simulink model "OneGFM_V2"  (R2020a)
settings: Solver=VariableStepAuto  StartTime=0.0  StopTime=10  RelTol=1e-6
InitFcn:
  | %initAll
values from neighbouring files (symbols this model uses):
  A_ = A(1:2*Ne,1:2*Ne) - B(1:2*Ne,1:2*Nu)/D(1:2*Nu,1:2*Nu)*C(1:2*Nu,1:2*Ne)    [init_V2.m]
  B_ = B(1:2*Ne,1:2*Nu)/D(1:2*Nu,1:2*Nu)    [init_V2.m]
  C_ = -D(1:2*Nu,1:2*Nu)\C(1:2*Nu,1:2*Ne)    [init_V2.m]
  D_ = inv(D(1:2*Nu,1:2*Nu))    [init_V2.m]
  GFMInit = GFM_init(opdata,GFM_in_gidx,SGFM)    [init_V2.m]
  Nu = length(G_in_gidx)    [init_V2.m]
  RG = gfmdata(:,3)    [GFL_init.m]    (also in GFM_init.m = gfmdata(:,3)./SGFM; GFMparaarea.m = 0; init_V2.m = 1e-06)
  VO = Vm(SG_in_gidx)+(opdata{num2str(SG_in_gidx),2}/1000-1i*opdata{num2str(SG_in_gidx),3}/1000)*RG    [init_V2.m]
  W0 = 2*pi*50    (= 314.159265359)    [GFMparaarea.m]    (also in ONEGFM_analysis.m = 314.1593; init_V2.m)
  X0 = -Adq\Bdq*udq    [init_V2.m]
undefined symbols (not defined in the file or in its folder): full, opdata
libraries: eeTransforms x4, simulink_extras x1
settings Model: Creator=LinSiQi  LastModifiedBy=Qiufan_Yang
settings DebuggingCC: ArithmeticOperatorsInVariantConditions=warning
settings SFSimCC: CustomCodeUndefinedFunction=UseInterfaceOnly
settings CodeAppCC: StateflowObjectComments=on
settings SimscapeCC: SimscapeNormalizeSystem=off

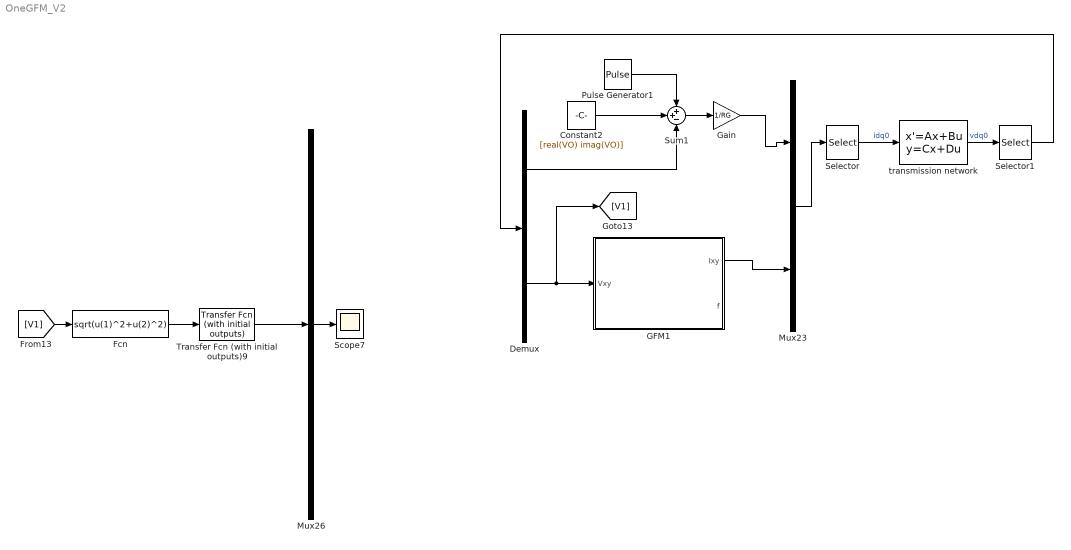
== system OneGFM_V2 ==
  Constant2 : Constant  Value=[real(VO) imag(VO)]
  Demux : Demux  Outputs=2
  Fcn : Fcn  Expr=sqrt(u(1)^2+u(2)^2)
  GFM1 : Subsystem  mask{Pout=opdata{1,2}, Qout=opdata{1,3}, Vout=opdata{1,4}*exp(1i*opdata{1,5}*pi/180), RG=GFMInit.RG(1), LG=GFMInit.LG(1), CF=GFMInit.CF(1), LF=GFMInit.LF(1), RF=GFMInit.RF(1), JGFM=GFMInit.J(1), DGFM=GFMInit.D(1), KPV=GFMInit.KPV(1), KIV=GFMInit.KIV(1), KIF=GFMInit.KIF(1), KPC=GFMInit.KPC(1), KIC=GFMInit.KIC(1), KVF=GFMInit.KVF(1), TVF=GFMInit.TVF(1), Pref=GFMInit.Pref(1), Qref=GFMInit.Qref(1), Vd0=GFMInit.Vd0(1), theta0=GFMInit.theta0(1), Ix0=GFMInit.Ix0(1), Iy0=GFMInit.Iy0(1), Vx0=GFMInit.Vx0(1), Vy0=GFMInit.Vy0(1), IOx0=GFMInit.IOx0(1), IOy0=GFMInit.IOy0(1), Idref0=GFMInit.Idref0(1), Iqref0=GFMInit.Iqref0(1), Ed0=GFMInit.Ed0(1), Eq0=GFMInit.Eq0(1)}
      mask init:
      | %IOxy0 = (Pout - 1i*Qout)/conj(Vout);
      | %Vxy0  = Vout + IOxy0*(RG+1i*LG);
      | %Ixy0  = IOxy0 + Vxy0*(1i*CF);
      | %Exy0  = Vxy0 + Ixy0*(RF+1i*LF);
      | 
      | %IOx0 = real(IOxy0);
      | % IOy0 = imag(IOxy0);
      | % Vx0 = real(Vxy0);
      | % Vy0 = imag(Vxy0);
      | % Ix0 = real(Ixy0);
      | % Iy0 = imag(Ixy0);
      | % Pref = real(Vxy0*conj(IOxy0));
      | % Qref = imag(Vxy0*conj(IOxy0));
      | % Vd0  = abs(Vxy0);
      | % theta0 = angle(Vxy0);
      | % 
      | % Edq0 = abs(Exy0)*exp(1i*(angle(Exy0)-theta0));
      | % Idq0 = abs(Ixy0)*exp(1i*(angle(Ixy0)-theta0));
      | % IOdq0 = abs(IOxy0)*exp(1i*(angle(IOxy0)-theta0));
      | % 
      | % temp = Edq0 - KVF*Vd0 - Idq0*(1i*LF);
      | % Ed0 = real(temp);
      | % Eq0 = imag(temp);
      | % 
      | % temp = Idq0 - KIF*IOdq0 - Vd0*(1i*CF);
      | % Idref0 = real(temp);
      | % Iqref0 = imag(temp);
      mask DialogControl Container8 Prompt: Parameters
      mask DialogControl Container9 Prompt: Power Flow
      mask DialogControl Container10 Prompt: LCL Parameters
      mask DialogControl Container20 Prompt: Control Parameters
      mask DialogControl Container21 Prompt: Initial Parameters
  Gain : Gain  Gain=1/RG
  Mux23 : Mux  Inputs=2
  Mux26 : Mux  Inputs=1
  Pulse Generator1 : DiscretePulseGenerator  PulseType=Time based  Amplitude=0.1  Period=10  PulseWidth=0.1  PhaseDelay=0.1
  Scope7 : Scope
  Selector : Selector  InputPortWidth=2*Nu  IndexOptions=Index vector (dialog)  Indices=units_to_net  OutputSizes=1
  Selector1 : Selector  InputPortWidth=2*Nu  IndexOptions=Index vector (dialog)  Indices=net_to_units  OutputSizes=1
  Sum1 : Sum  Inputs=++-
  Transfer Fcn (with initial outputs)9 : simulink_extras/Additional Linear/Transfer Fcn (with initial outputs)  N=[1]  D="[0.001  1]"  Y0=opdata{1,4}  U0=opdata{1,4}
  transmission network : StateSpace  A=full(A_)  B=full(B_)  C=full(C_)  D=full(D_)  InitialCondition=X0
  wires:
  Mux23/1 -> Selector/1
  transmission network/1 -> Selector1/1  "vdq0"
  Selector/1 -> transmission network/1  "idq0"
  Mux26/1 -> Scope7/1
  [V1] -> Fcn/1
  Fcn/1 -> Transfer Fcn (with initial outputs)9/1
  Transfer Fcn (with initial outputs)9/1 -> Mux26/1
  Demux/2 -> [V1], GFM1/1(Vxy)
  GFM1/1(Ixy) -> Mux23/2
  Selector1/1 -> Demux/1
  Sum1/1 -> Gain/1
  Constant2/1 -> Sum1/2
  Pulse Generator1/1 -> Sum1/1
  Demux/1 -> Sum1/3
  Gain/1 -> Mux23/1

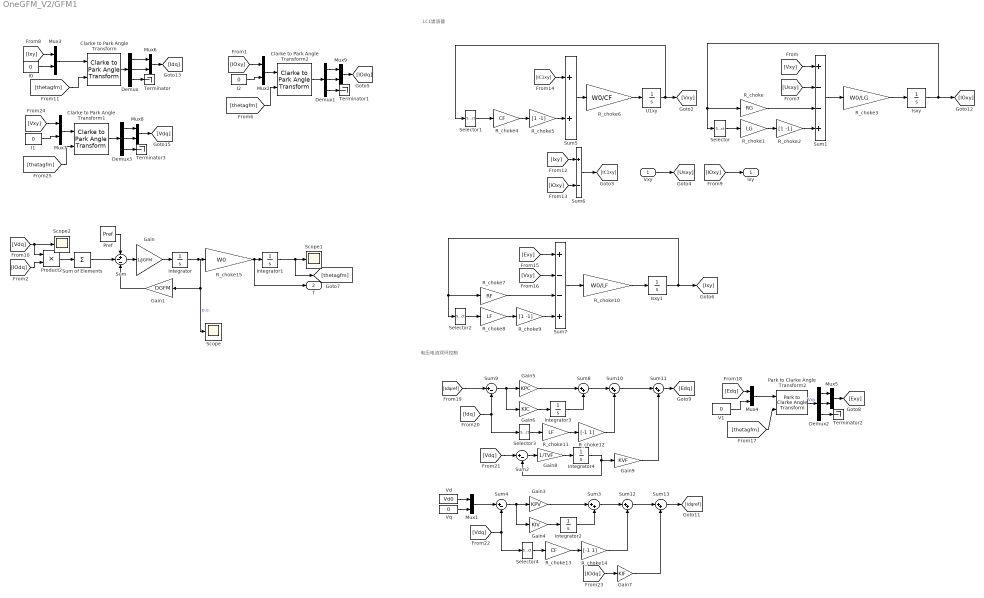
== system OneGFM_V2/GFM1 ==
  note: 电压电流双环控制
  note: LCL滤波器
  Vxy : Inport
  Clarke to Park Angle Transform : eeTransforms/Clarke to Park Angle Transform  AxisAlignment=D-axis
      settings: SourceProductBaseCode=PS
  Clarke to Park Angle Transform1 : eeTransforms/Clarke to Park Angle Transform  AxisAlignment=D-axis
      settings: SourceProductBaseCode=PS
  Clarke to Park Angle Transform2 : eeTransforms/Clarke to Park Angle Transform  AxisAlignment=D-axis
      settings: SourceProductBaseCode=PS
  Demux{,1..3} (4 alike) : Demux  Outputs=3
  Gain : Gain  Gain=1/JGFM
  Gain1 : Gain  Gain=DGFM
  Gain3 : Gain  Gain=KPV
  Gain4 : Gain  Gain=KIV
  Gain5 : Gain  Gain=KPC
  Gain6 : Gain  Gain=KIC
  Gain7 : Gain  Gain=KIF
  Gain8 : Gain  Gain=1/TVF
  Gain9 : Gain  Gain=KVF
  I0 : Constant  Value=0
  I1 : Constant  Value=0
  I2 : Constant  Value=0
  Integrator : Integrator
  Integrator1 : Integrator  InitialCondition=theta0
  Integrator2 : Integrator  InitialCondition=[Idref0 Iqref0]
  Integrator3 : Integrator  InitialCondition=[Ed0 Eq0]
  Integrator4 : Integrator  InitialCondition=[Vd0 0]
  Isxy : Integrator  InitialCondition=[IOx0 IOy0]
  Isxy1 : Integrator  InitialCondition=[Ix0 Iy0]
  Mux{1..9} (9 alike) : Mux  Inputs=2
  Park to Clarke Angle Transform2 : eeTransforms/Park to Clarke Angle Transform  AxisAlignment=D-axis
      settings: SourceProductBaseCode=PS
  Pref : Constant  Value=Pref
  Product2 : Product
  R_choke : Gain  Gain=RG  SaturateOnIntegerOverflow=on  OutDataTypeStr=Inherit: Same as input  ParamDataTypeStr=Inherit: Same as input
  R_choke1 : Gain  Gain=LG  SaturateOnIntegerOverflow=on  OutDataTypeStr=Inherit: Same as input  ParamDataTypeStr=Inherit: Same as input
  R_choke10 : Gain  Gain=W0/LF  SaturateOnIntegerOverflow=on  OutDataTypeStr=Inherit: Same as input  ParamDataTypeStr=Inherit: Same as input
  R_choke11 : Gain  Gain=LF  SaturateOnIntegerOverflow=on  OutDataTypeStr=Inherit: Same as input  ParamDataTypeStr=Inherit: Same as input
  R_choke12 : Gain  Gain=[-1 1]  SaturateOnIntegerOverflow=on  OutDataTypeStr=Inherit: Same as input  ParamDataTypeStr=Inherit: Same as input
  R_choke13 : Gain  Gain=CF  SaturateOnIntegerOverflow=on  OutDataTypeStr=Inherit: Same as input  ParamDataTypeStr=Inherit: Same as input
  R_choke14 : Gain  Gain=[-1 1]  SaturateOnIntegerOverflow=on  OutDataTypeStr=Inherit: Same as input  ParamDataTypeStr=Inherit: Same as input
  R_choke15 : Gain  Gain=W0  SaturateOnIntegerOverflow=on  OutDataTypeStr=Inherit: Same as input  ParamDataTypeStr=Inherit: Same as input
  R_choke2 : Gain  Gain=[1 -1]  SaturateOnIntegerOverflow=on  OutDataTypeStr=Inherit: Same as input  ParamDataTypeStr=Inherit: Same as input
  R_choke3 : Gain  Gain=W0/LG  SaturateOnIntegerOverflow=on  OutDataTypeStr=Inherit: Same as input  ParamDataTypeStr=Inherit: Same as input
  R_choke4 : Gain  Gain=CF  SaturateOnIntegerOverflow=on  OutDataTypeStr=Inherit: Same as input  ParamDataTypeStr=Inherit: Same as input
  R_choke5 : Gain  Gain=[1 -1]  SaturateOnIntegerOverflow=on  OutDataTypeStr=Inherit: Same as input  ParamDataTypeStr=Inherit: Same as input
  R_choke6 : Gain  Gain=W0/CF  SaturateOnIntegerOverflow=on  OutDataTypeStr=Inherit: Same as input  ParamDataTypeStr=Inherit: Same as input
  R_choke7 : Gain  Gain=RF  SaturateOnIntegerOverflow=on  OutDataTypeStr=Inherit: Same as input  ParamDataTypeStr=Inherit: Same as input
  R_choke8 : Gain  Gain=LF  SaturateOnIntegerOverflow=on  OutDataTypeStr=Inherit: Same as input  ParamDataTypeStr=Inherit: Same as input
  R_choke9 : Gain  Gain=[1 -1]  SaturateOnIntegerOverflow=on  OutDataTypeStr=Inherit: Same as input  ParamDataTypeStr=Inherit: Same as input
  Scope : Scope
  Scope1 : Scope
  Scope2 : Scope
  Selector{,1..4} (5 alike) : Selector  InputPortWidth=2  IndexOptions=Index vector (dialog)  Indices=[2 1]  OutputSizes=1
  Sum : Sum  Inputs=+--
  Sum of Elements : Sum  Inputs=+
  Sum1 : Sum  Inputs=+--+  SaturateOnIntegerOverflow=on
  Sum{3,8,10..13} (6 alike) : Sum  Inputs=|++
  Sum2 : Sum  Inputs=|+-
  Sum4 : Sum  Inputs=|+-
  Sum5 : Sum  SaturateOnIntegerOverflow=on
  Sum6 : Sum  Inputs=+-  SaturateOnIntegerOverflow=on
  Sum7 : Sum  Inputs=+--+  SaturateOnIntegerOverflow=on
  Sum9 : Sum  Inputs=|+-
  Terminator{,1..3} (4 alike) : Terminator
  U1xy : Integrator  InitialCondition=[Vx0 Vy0]
  V1 : Constant  Value=0
  Vd : Constant  Value=Vd0
  Vq : Constant  Value=0
  Ixy : Outport
  f : Outport  Port=2
  wires:
  Gain1/1 -> Sum/3
  Integrator1/1 -> [thetagfm], Scope1/1
  Mux3/1 -> Clarke to Park Angle Transform/1
  I0/1 -> Mux3/2
  Demux/3 -> Terminator/1
  Demux/2 -> Mux6/2
  Gain/1 -> Integrator/1
  Demux/1 -> Mux6/1
  Clarke to Park Angle Transform/1 -> Demux/1
  Integrator/1 -> Scope/1, Gain1/1, R_choke15/1  "p.u."
  Sum of Elements/1 -> Sum/2
  Sum/1 -> Gain/1
  Vxy/1 -> [Usxy]
  [Vxy] -> Sum1/1
  [Usxy] -> Sum1/2
  Sum1/1 -> R_choke3/1
  R_choke3/1 -> Isxy/1
  R_choke1/1 -> R_choke2/1
  Isxy/1 -> [IOxy], R_choke/1, Selector/1
  R_choke/1 -> Sum1/3
  Selector/1 -> R_choke1/1
  R_choke2/1 -> Sum1/4
  [Ixy] -> Mux3/1
  [IOxy] -> Ixy/1
  [thetagfm] -> Clarke to Park Angle Transform/2
  Gain4/1 -> Integrator2/1
  Sum3/1 -> Sum12/1
  Gain3/1 -> Sum3/1
  Integrator2/1 -> Sum3/2
  Sum4/1 -> Gain4/1, Gain3/1
  Vd/1 -> Mux1/1
  Vq/1 -> Mux1/2
  Mux1/1 -> Sum4/1
  R_choke4/1 -> R_choke5/1
  R_choke5/1 -> Sum5/2
  Sum6/1 -> [IC1xy]
  U1xy/1 -> Selector1/1, [Vxy]
  R_choke6/1 -> U1xy/1
  [Ixy] -> Sum6/1
  Selector1/1 -> R_choke4/1
  [IOxy] -> Sum6/2
  [IC1xy] -> Sum5/1
  Sum5/1 -> R_choke6/1
  Isxy1/1 -> [Ixy], R_choke7/1, Selector2/1
  [Vxy] -> Sum7/2
  R_choke7/1 -> Sum7/3
  R_choke8/1 -> R_choke9/1
  R_choke10/1 -> Isxy1/1
  Sum7/1 -> R_choke10/1
  R_choke9/1 -> Sum7/4
  Selector2/1 -> R_choke8/1
  [Edq] -> Mux4/1
  V1/1 -> Mux4/2
  Mux4/1 -> Park to Clarke Angle Transform2/1
  [thetagfm] -> Park to Clarke Angle Transform2/2
  Mux5/1 -> [Exy]
  Demux2/3 -> Terminator2/1
  Park to Clarke Angle Transform2/1 -> Demux2/1  "Vxy"
  Demux2/2 -> Mux5/2
  Demux2/1 -> Mux5/1
  [Idqref] -> Sum9/1
  Sum9/1 -> Gain6/1, Gain5/1
  Gain5/1 -> Sum8/1
  Gain6/1 -> Integrator3/1
  Integrator3/1 -> Sum8/2
  [Idq] -> Sum9/2, Selector3/1
  R_choke11/1 -> R_choke12/1
  Selector3/1 -> R_choke11/1
  Sum8/1 -> Sum10/1
  R_choke12/1 -> Sum10/2
  Sum10/1 -> Sum11/1
  Gain9/1 -> Sum11/2
  Sum11/1 -> [Edq]
  Selector4/1 -> R_choke13/1
  [Vdq] -> Selector4/1, Sum4/2
  R_choke13/1 -> R_choke14/1
  R_choke14/1 -> Sum12/2
  Sum12/1 -> Sum13/1
  Sum13/1 -> [Idqref]
  [IOdq] -> Gain7/1
  Gain7/1 -> Sum13/2
  Mux6/1 -> [Idq]
  [Vxy] -> Mux7/1
  I1/1 -> Mux7/2
  Mux7/1 -> Clarke to Park Angle Transform1/1
  [thetagfm] -> Clarke to Park Angle Transform1/2
  Clarke to Park Angle Transform1/1 -> Demux3/1
  Demux3/1 -> Mux8/1
  Demux3/2 -> Mux8/2
  Mux8/1 -> [Vdq]
  Demux3/3 -> Terminator3/1
  [thetagfm] -> Clarke to Park Angle Transform2/2
  Clarke to Park Angle Transform2/1 -> Demux1/1
  Demux1/1 -> Mux9/1
  Demux1/2 -> Mux9/2
  [IOxy] -> Mux2/1
  Demux1/3 -> Terminator1/1
  Mux2/1 -> Clarke to Park Angle Transform2/1
  Mux9/1 -> [IOdq]
  I2/1 -> Mux2/2
  [Vdq] -> Scope2/1, Product2/1
  [IOdq] -> Product2/2
  Product2/1 -> Sum of Elements/1
  Sum2/1 -> Gain8/1
  Integrator4/1 -> Gain9/1, Sum2/2
  Gain8/1 -> Integrator4/1
  [Vdq] -> Sum2/1
  [Exy] -> Sum7/1
  Pref/1 -> Sum/1
  R_choke15/1 -> f/1, Integrator1/1
